simulink model "exampleStartDelay"  (Simulink 7.6)
settings: Solver=ode45  StartTime=0.0  StopTime=30  RelTol=1e-3
settings Model: Creator=drhf  LastModifiedBy=awohlfei
settings CodeAppCC: CustomSymbolStrType=$N$R$M_T

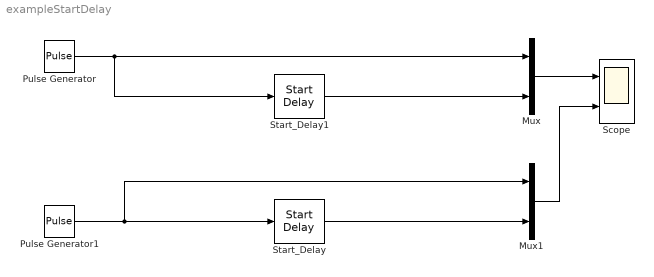
== system exampleStartDelay ==
  Mux : Mux  Inputs=2
  Mux1 : Mux  Inputs=2
  Pulse Generator : DiscretePulseGenerator  PulseType=Time based  Amplitude=2  Period=10  PulseWidth=10
  Pulse Generator1 : DiscretePulseGenerator  PulseType=Time based  Amplitude=2  Period=10  PulseWidth=80
  Scope : Scope  NumInputPorts=2
      settings: YMin=-5~-5  YMax=5~5
  Start_Delay : Reference  SystemSampleTime=-1  tstartdelay=5
  Start_Delay1 : Reference  SystemSampleTime=-1  tstartdelay=5
  wires:
  Pulse Generator/1 -> Mux/1, Start_Delay1/1
  Mux/1 -> Scope/1
  Start_Delay1/1 -> Mux/2
  Pulse Generator1/1 -> Mux1/1, Start_Delay/1
  Start_Delay/1 -> Mux1/2
  Mux1/1 -> Scope/2
